simulink model "controller_template"  (Simulink 8.1)
settings: Solver=ode3  SolverMode=SingleTasking  StartTime=0.0  StopTime=inf  FixedStep=Ts  RelTol=1e-3
PreLoadFcn:
  | load_waypoints
values from neighbouring files (symbols this model uses):
  g = 9.8065    [kostas_malakies.mat]    (also in kostas_malakies2.mat; load_PMModel.m = 9.81; main.m; main_last.m)
  pitch_cmd2pitch_1stOrd = 1.42468924998    [kostas_malakies.mat]    (also in kostas_malakies2.mat)
  roll_cmd2roll_1stOrd = 1.38101661575    [kostas_malakies.mat]    (also in kostas_malakies2.mat)
  thrust_cmd2thrust_0thOrd = 0.876575459522    [kostas_malakies.mat]    (also in kostas_malakies2.mat)
  THRUST_CMD_GAIN = -0.0835    [kostas_malakies.mat]    (also in kostas_malakies2.mat; load_PMModel.m)
  yaw_cmd2yaw_1stOrd = 2.01792090263    [kostas_malakies.mat]    (also in kostas_malakies2.mat)
  z = [-0.93079906702 -0.933865725994 -0.937557637691 -0.939011216164 -0.94143640995 -0.944628417492 -0.947235524654 -0.949601888657 -0.952827751637 -0.9567258358 -0.958320975304 -0.960991024971 ... (7988 elements, 7988x1)]    [kostas_malakies2.mat]    (also in plotDataTest.m = simout_data.signals.values(:,11))
libraries: Hquad_control_LIB_MPC x3, simulink x1
settings Model: Creator=janosch  LastModifiedBy=burrimi  SimulationMode=external
settings DataIOCC: SaveOutput=off  SaveTime=off
settings OptimizationCC: OptimizeModelRefInitCode=on  LifeSpan=Inf
settings DebuggingCC: ParameterPrecisionLossMsg=none
settings HardwareCC: ProdIntDivRoundTo=Zero  ProdEndianess=LittleEndian  ProdHWDeviceType=Intel Pentium
settings RTWCC: SystemTargetFile=ert.tlc  TemplateMakefile=ert_default_tmf  Description=Embedded Coder  ProcessScript=ert_make_rtw_hook  CustomHeaderCode=#include <math.h>  TargetLang=C++  RTWCompilerOptimization=On
settings CodeAppCC: IgnoreCustomStorageClasses=off  CustomSymbolStrType=$N$R$M  InternalIdentifier=Classic
settings ERTTargetCC: CodeReplacementLibrary=ANSI_C  MultiwordLength=2048  GenerateSampleERTMain=on  SupportNonInlinedSFcns=on  ExtMode=on  ERTCustomFileTemplate=example_file_process.tlc  ConvertIfToSwitch=off  SuppressUnreachableDefaultCases=off
settings ConfigurationSet: Description=SimMechanics 2G

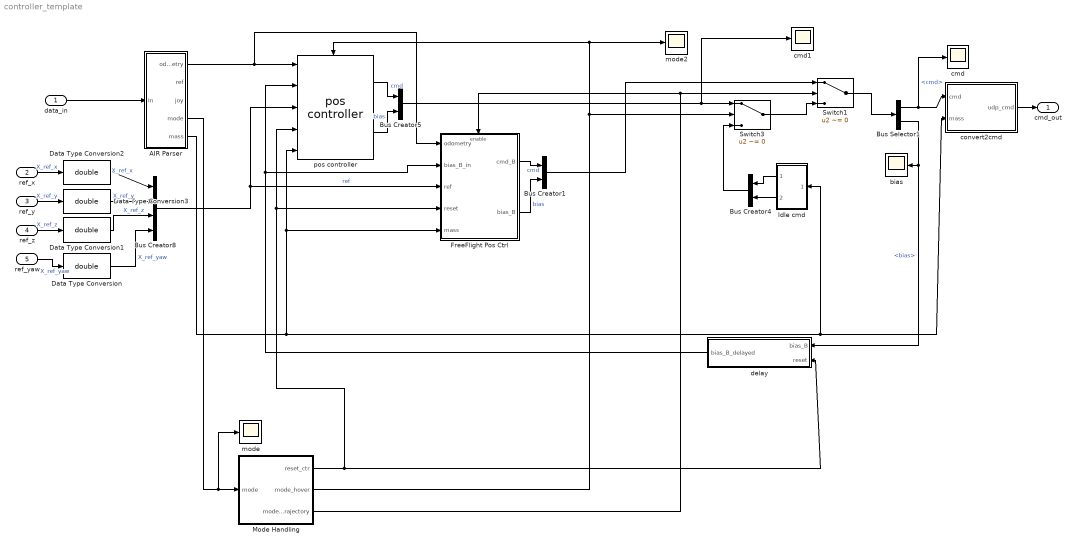
== system controller_template ==
  data_in : Inport  OutDataTypeStr=single  PortDimensions=30
  ref_x : Inport  Port=2  OutDataTypeStr=single  PortDimensions=93
  ref_y : Inport  Port=3  OutDataTypeStr=single  PortDimensions=93
  ref_z : Inport  Port=4  OutDataTypeStr=single  PortDimensions=62
  ref_yaw : Inport  Port=5  OutDataTypeStr=single  PortDimensions=62
  AIR Parser : Subsystem
  Bus Creator1 : BusCreator  Inputs=2
  Bus Creator4 : BusCreator  Inputs=2
  Bus Creator5 : BusCreator  Inputs=2
  Bus Creator8 : BusCreator
  Bus Selector1 : BusSelector  OutputSignals=cmd,bias
  Data Type Conversion{,1..3} (4 alike) : DataTypeConversion  OutDataTypeStr=double
  FreeFlight Pos Ctrl : Subsystem  AncestorBlock=Hquad_control_LIB_MPC/pos controller
  Idle cmd : Subsystem
  Mode Handling : Subsystem
  Switch1 : Switch  Criteria=u2 ~= 0
  Switch3 : Switch  Criteria=u2 ~= 0
  bias : Scope
      settings: TickLabels=on  TimeRange=40  YMin=-0.3  YMax=0.075  SaveName=ScopeData9
  cmd : Scope
      settings: YMin=-0.5  YMax=7  SaveName=ScopeData4
  cmd1 : Scope
      settings: YMin=-0.5  YMax=7  SaveName=ScopeData15
  convert2cmd : Subsystem
  delay : Subsystem
  mode : Scope
      settings: YMin=0  YMax=6  SaveName=ScopeData6
  mode2 : Scope
      settings: YMin=0  YMax=6  SaveName=ScopeData14
  pos controller : Hquad_control_LIB_MPC/pos controller
  cmd_out : Outport  PortDimensions=4
  wires:
  Mode Handling/1(reset_ctr) -> delay/2(reset), pos controller/4, FreeFlight Pos Ctrl/4(reset)
  Mode Handling/2(mode_hover) -> Switch3/2, mode2/1, pos controller/Enable
  AIR Parser/4(mode) -> mode/1, Mode Handling/1(mode)
  Bus Creator5/1 -> Switch3/1, cmd1/1
  pos controller/1 -> Bus Creator5/1  "cmd"
  pos controller/2 -> Bus Creator5/2  "bias"
  Bus Selector1/1 -> convert2cmd/1(cmd), cmd/1  "<cmd>"
  Bus Selector1/2 -> bias/1, delay/1(bias_B)  "<bias>"
  delay/1(bias_B_delayed) -> FreeFlight Pos Ctrl/2(bias_B_in), pos controller/2
  convert2cmd/1(udp_cmd) -> cmd_out/1
  data_in/1 -> AIR Parser/1(In)
  Idle cmd/1(cmd) -> Bus Creator4/1
  Idle cmd/2(bias) -> Bus Creator4/2
  Bus Creator4/1 -> Switch3/3
  AIR Parser/1(odometry) -> FreeFlight Pos Ctrl/1(odometry), pos controller/1
  ref_x/1 -> Data Type Conversion2/1  "X_ref_x"
  ref_y/1 -> Data Type Conversion3/1  "X_ref_y"
  ref_z/1 -> Data Type Conversion1/1  "X_ref_z"
  ref_yaw/1 -> Data Type Conversion/1  "X_ref_yaw"
  Data Type Conversion/1 -> Bus Creator8/4  "X_ref_yaw"
  Data Type Conversion1/1 -> Bus Creator8/3  "X_ref_z"
  Data Type Conversion2/1 -> Bus Creator8/1  "X_ref_x"
  Data Type Conversion3/1 -> Bus Creator8/2  "X_ref_y"
  Switch3/1 -> Switch1/3
  Switch1/1 -> Bus Selector1/1
  Mode Handling/3(mode_trajectory) -> FreeFlight Pos Ctrl/Enable, Switch1/2
  AIR Parser/5(mass) -> Idle cmd/1(mass), convert2cmd/2(mass), pos controller/5, FreeFlight Pos Ctrl/5(mass)
  Bus Creator8/1 -> pos controller/3, FreeFlight Pos Ctrl/3(ref)  "ref"
  Bus Creator1/1 -> Switch1/1
  FreeFlight Pos Ctrl/1(cmd_B) -> Bus Creator1/1  "cmd"
  FreeFlight Pos Ctrl/2(bias_B) -> Bus Creator1/2  "bias"

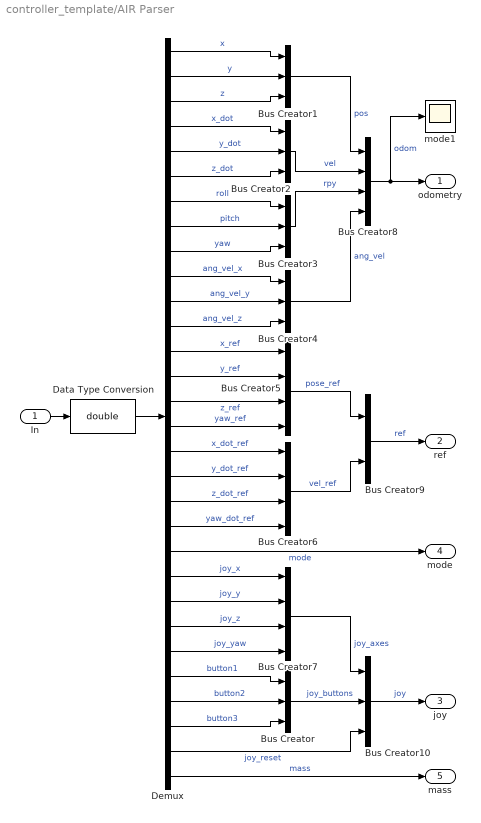
== system controller_template/AIR Parser ==
  In : Inport
  Bus Creator{,1..4,10} (6 alike) : BusCreator  Inputs=3
  Bus Creator{5..8} (4 alike) : BusCreator
  Bus Creator9 : BusCreator  Inputs=2
  Data Type Conversion : DataTypeConversion  OutDataTypeStr=double
  Demux : Demux  Outputs=30
  mode1 : Scope
      settings: YMin=0  YMax=6  SaveName=ScopeData7
  odometry : Outport
  ref : Outport  Port=2
  joy : Outport  Port=3
  mode : Outport  Port=4
  mass : Outport  Port=5
  wires:
  In/1 -> Data Type Conversion/1
  Data Type Conversion/1 -> Demux/1
  Demux/1 -> Bus Creator1/1  "x"
  Demux/7 -> Bus Creator3/1  "roll"
  Demux/8 -> Bus Creator3/2  "pitch"
  Demux/9 -> Bus Creator3/3  "yaw"
  Demux/15 -> Bus Creator5/3  "z_ref"
  Demux/14 -> Bus Creator5/2  "y_ref"
  Demux/13 -> Bus Creator5/1  "x_ref"
  Demux/16 -> Bus Creator5/4  "yaw_ref"
  Demux/2 -> Bus Creator1/2  "y"
  Demux/3 -> Bus Creator1/3  "z"
  Demux/4 -> Bus Creator2/1  "x_dot"
  Demux/5 -> Bus Creator2/2  "y_dot"
  Demux/6 -> Bus Creator2/3  "z_dot"
  Demux/19 -> Bus Creator6/3  "z_dot_ref"
  Demux/18 -> Bus Creator6/2  "y_dot_ref"
  Demux/17 -> Bus Creator6/1  "x_dot_ref"
  Demux/20 -> Bus Creator6/4  "yaw_dot_ref"
  Demux/12 -> Bus Creator4/3  "ang_vel_z"
  Demux/11 -> Bus Creator4/2  "ang_vel_y"
  Demux/10 -> Bus Creator4/1  "ang_vel_x"
  Demux/21 -> mode/1  "mode"
  Bus Creator5/1 -> Bus Creator9/1  "pose_ref"
  Bus Creator6/1 -> Bus Creator9/2  "vel_ref"
  Demux/22 -> Bus Creator7/1  "joy_x"
  Demux/23 -> Bus Creator7/2  "joy_y"
  Demux/24 -> Bus Creator7/3  "joy_z"
  Demux/25 -> Bus Creator7/4  "joy_yaw"
  Bus Creator7/1 -> Bus Creator10/1  "joy_axes"
  Demux/26 -> Bus Creator/1  "button1"
  Demux/28 -> Bus Creator/3  "button3"
  Demux/27 -> Bus Creator/2  "button2"
  Bus Creator/1 -> Bus Creator10/2  "joy_buttons"
  Bus Creator4/1 -> Bus Creator8/4  "ang_vel"
  Bus Creator3/1 -> Bus Creator8/3  "rpy"
  Bus Creator2/1 -> Bus Creator8/2  "vel"
  Bus Creator1/1 -> Bus Creator8/1  "pos"
  Demux/29 -> Bus Creator10/3  "joy_reset"
  Bus Creator10/1 -> joy/1  "joy"
  Bus Creator9/1 -> ref/1  "ref"
  Bus Creator8/1 -> odometry/1, mode1/1  "odom"
  Demux/30 -> mass/1  "mass"

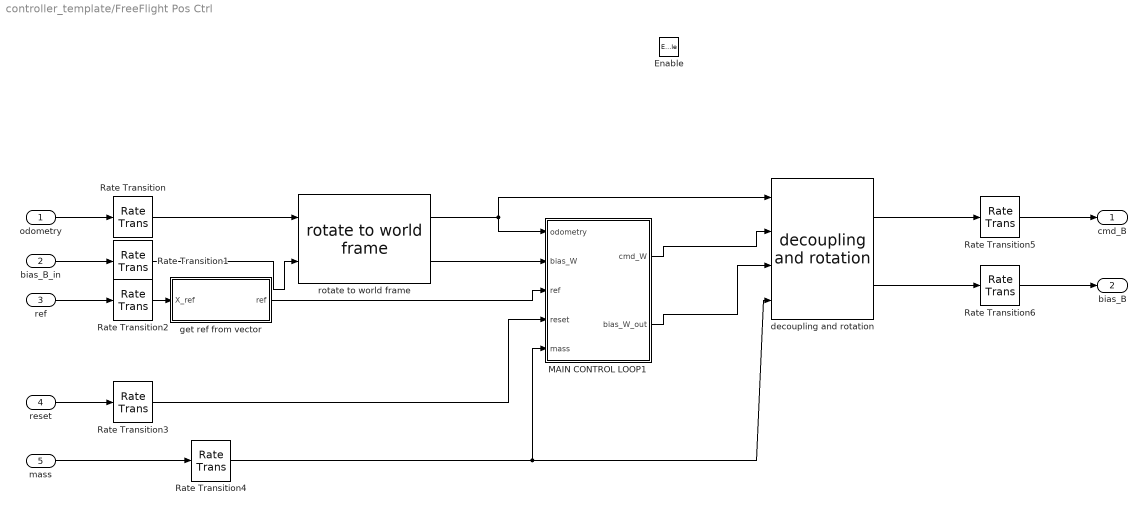
== system controller_template/FreeFlight Pos Ctrl ==
  odometry : Inport
  bias_B_in : Inport  Port=2
  ref : Inport  Port=3
  reset : Inport  Port=4
  mass : Inport  Port=5
  Enable : EnablePort  StatesWhenEnabling=reset
  MAIN CONTROL LOOP1 : Subsystem  Priority=2  AncestorBlock=Hquad_control_LIB_MPC/MAIN CONTROL LOOP  TreatAsAtomicUnit=on
  Rate Transition{,1..4} (5 alike) : RateTransition  OutPortSampleTime=0.08
  Rate Transition5 : RateTransition  OutPortSampleTime=Ts
  Rate Transition6 : RateTransition  OutPortSampleTime=Ts
  decoupling and rotation : Hquad_control_LIB_MPC/decoupling and rotation  Priority=3
  get ref from vector : Subsystem
  rotate to world frame : Hquad_control_LIB_MPC/rotate to world frame  Priority=1
  cmd_B : Outport
  bias_B : Outport  Port=2
  wires:
  mass/1 -> Rate Transition4/1
  bias_B_in/1 -> Rate Transition1/1
  rotate to world frame/2 -> MAIN CONTROL LOOP1/2(bias_W)
  decoupling and rotation/2 -> Rate Transition6/1
  decoupling and rotation/1 -> Rate Transition5/1
  MAIN CONTROL LOOP1/2(bias_W_out) -> decoupling and rotation/3
  rotate to world frame/1 -> decoupling and rotation/1, MAIN CONTROL LOOP1/1(odometry)
  ref/1 -> Rate Transition2/1
  reset/1 -> Rate Transition3/1
  MAIN CONTROL LOOP1/1(cmd_W) -> decoupling and rotation/2
  odometry/1 -> Rate Transition/1
  get ref from vector/1(ref) -> MAIN CONTROL LOOP1/3(ref)
  Rate Transition/1 -> rotate to world frame/1
  Rate Transition1/1 -> rotate to world frame/2
  Rate Transition2/1 -> get ref from vector/1(X_ref)
  Rate Transition3/1 -> MAIN CONTROL LOOP1/4(reset)
  Rate Transition4/1 -> decoupling and rotation/4, MAIN CONTROL LOOP1/5(mass)
  Rate Transition5/1 -> cmd_B/1
  Rate Transition6/1 -> bias_B/1

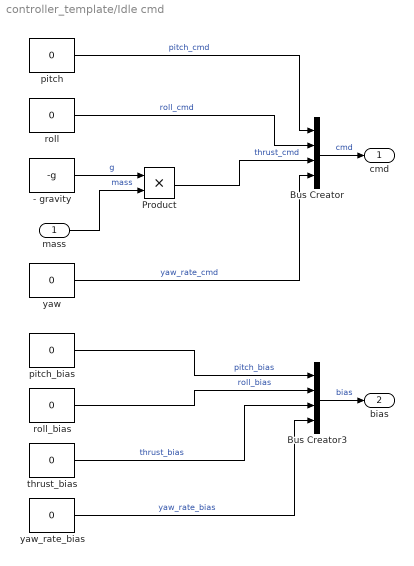
== system controller_template/Idle cmd ==
  mass : Inport  OutDataTypeStr=double
  - gravity : Constant  Value=-g
  Bus Creator : BusCreator
  Bus Creator3 : BusCreator
  Product : Product  RndMeth=Zero
  pitch : Constant  Value=0
  pitch_bias : Constant  Value=0
  roll : Constant  Value=0
  roll_bias : Constant  Value=0
  thrust_bias : Constant  Value=0
  yaw : Constant  Value=0
  yaw_rate_bias : Constant  Value=0
  cmd : Outport
  bias : Outport  Port=2
  wires:
  roll/1 -> Bus Creator/2  "roll_cmd"
  pitch/1 -> Bus Creator/1  "pitch_cmd"
  Bus Creator/1 -> cmd/1  "cmd"
  yaw/1 -> Bus Creator/4  "yaw_rate_cmd"
  pitch_bias/1 -> Bus Creator3/1  "pitch_bias"
  roll_bias/1 -> Bus Creator3/2  "roll_bias"
  thrust_bias/1 -> Bus Creator3/3  "thrust_bias"
  yaw_rate_bias/1 -> Bus Creator3/4  "yaw_rate_bias"
  Bus Creator3/1 -> bias/1  "bias"
  - gravity/1 -> Product/1  "g"
  Product/1 -> Bus Creator/3  "thrust_cmd"
  mass/1 -> Product/2  "mass"

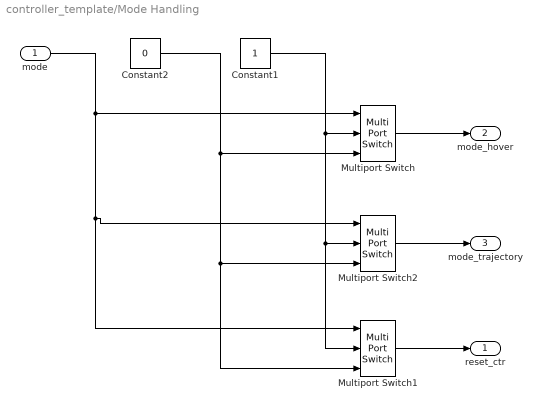
== system controller_template/Mode Handling ==
  mode : Inport
  Constant1 : Constant
  Constant2 : Constant  Value=0
  Multiport Switch : MultiPortSwitch  DataPortOrder=Specify indices  Inputs=2  DataPortIndices={[1,2,3],0}
  Multiport Switch1 : MultiPortSwitch  DataPortOrder=Specify indices  Inputs=2  DataPortIndices={[10],0}
  Multiport Switch2 : MultiPortSwitch  DataPortOrder=Specify indices  Inputs=2  DataPortIndices={[4],0}
  reset_ctr : Outport
  mode_hover : Outport  Port=2
  mode_trajectory : Outport  Port=3
  wires:
  Constant1/1 -> Multiport Switch/2, Multiport Switch1/2, Multiport Switch2/2
  Constant2/1 -> Multiport Switch/3, Multiport Switch1/3, Multiport Switch2/3
  Multiport Switch1/1 -> reset_ctr/1
  mode/1 -> Multiport Switch/1, Multiport Switch1/1, Multiport Switch2/1
  Multiport Switch/1 -> mode_hover/1
  Multiport Switch2/1 -> mode_trajectory/1

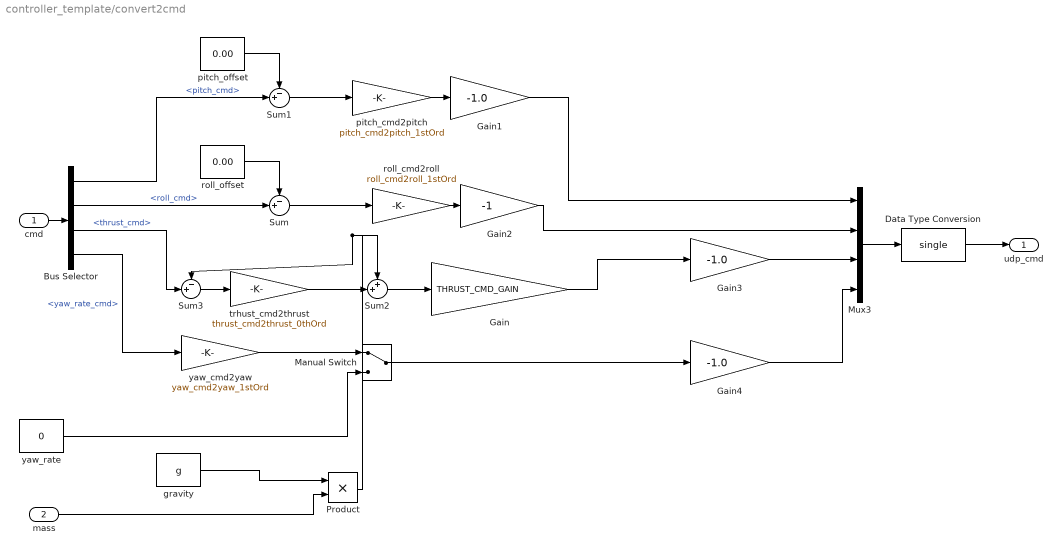
== system controller_template/convert2cmd ==
  cmd : Inport
  mass : Inport  Port=2
  Bus Selector : BusSelector  OutputSignals=pitch_cmd,roll_cmd,thrust_cmd,yaw_rate_cmd
  Data Type Conversion : DataTypeConversion  OutDataTypeStr=single
  Gain : Gain  Gain=THRUST_CMD_GAIN
  Gain1 : Gain  Gain=-1.0
  Gain2 : Gain  Gain=-1
  Gain3 : Gain  Gain=-1.0
  Gain4 : Gain  Gain=-1.0
  Manual Switch : ManualSwitch
  Mux3 : Mux
  Product : Product  RndMeth=Zero
  Sum : Sum  Inputs=-+|
  Sum1 : Sum  Inputs=-+|
  Sum2 : Sum  Inputs=++|
  Sum3 : Sum  Inputs=-+|
  gravity : Constant  Value=g
  pitch_cmd2pitch : Gain  Gain=pitch_cmd2pitch_1stOrd
  pitch_offset : Constant  Value=0.00
  roll_cmd2roll : Gain  Gain=roll_cmd2roll_1stOrd
  roll_offset : Constant  Value=0.00
  trhust_cmd2thrust : Gain  Gain=thrust_cmd2thrust_0thOrd
  yaw_cmd2yaw : Gain  Gain=yaw_cmd2yaw_1stOrd
  yaw_rate : Constant  Value=0
  udp_cmd : Outport
  wires:
  pitch_cmd2pitch/1 -> Gain1/1
  Bus Selector/2 -> Sum/2  "<roll_cmd>"
  Sum/1 -> roll_cmd2roll/1
  roll_offset/1 -> Sum/1
  Gain4/1 -> Mux3/4
  Gain3/1 -> Mux3/3
  Gain2/1 -> Mux3/2
  Gain/1 -> Gain3/1
  Gain1/1 -> Mux3/1
  pitch_offset/1 -> Sum1/1
  Sum1/1 -> pitch_cmd2pitch/1
  Mux3/1 -> Data Type Conversion/1
  Data Type Conversion/1 -> udp_cmd/1
  Product/1 -> Sum2/1, Sum3/1
  Sum2/1 -> Gain/1
  Manual Switch/1 -> Gain4/1
  yaw_rate/1 -> Manual Switch/2
  cmd/1 -> Bus Selector/1
  Bus Selector/1 -> Sum1/2  "<pitch_cmd>"
  yaw_cmd2yaw/1 -> Manual Switch/1
  trhust_cmd2thrust/1 -> Sum2/2
  roll_cmd2roll/1 -> Gain2/1
  Bus Selector/3 -> Sum3/2  "<thrust_cmd>"
  Sum3/1 -> trhust_cmd2thrust/1
  Bus Selector/4 -> yaw_cmd2yaw/1  "<yaw_rate_cmd>"
  gravity/1 -> Product/1
  mass/1 -> Product/2

== system controller_template/delay ==
  bias_B : Inport
  reset : Inport  Port=2
  Bus Creator1 : BusCreator
  Demux1 : Demux
  delay bias : simulink/Additional Math & Discrete/Additional Discrete/Unit Delay Resettable  vinit=0.0  tsamp=-1
  bias_B_delayed : Outport
  wires:
  Demux1/1 -> Bus Creator1/1  "pitch_bias"
  Demux1/2 -> Bus Creator1/2  "roll_bias"
  Demux1/3 -> Bus Creator1/3  "thrust_bias"
  Demux1/4 -> Bus Creator1/4  "yaw_rate_bias"
  delay bias/1 -> Demux1/1
  bias_B/1 -> delay bias/1
  reset/1 -> delay bias/2
  Bus Creator1/1 -> bias_B_delayed/1

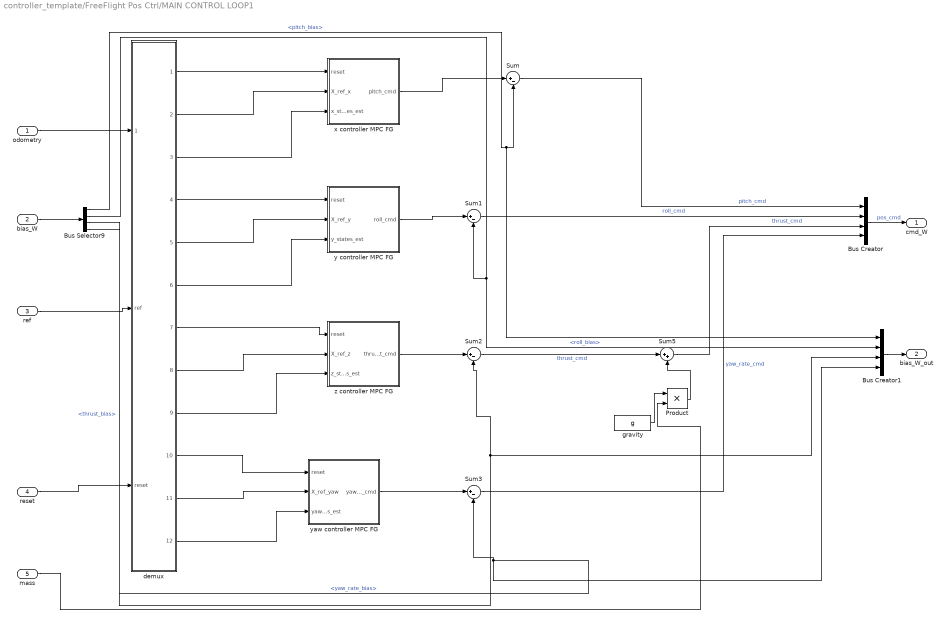
== system controller_template/FreeFlight Pos Ctrl/MAIN CONTROL LOOP1 ==
  odometry : Inport
  bias_W : Inport  Port=2
  ref : Inport  Port=3
  reset : Inport  Port=4
  mass : Inport  Port=5
  Bus Creator : BusCreator
  Bus Creator1 : BusCreator
  Bus Selector9 : BusSelector  OutputSignals=pitch_bias,roll_bias,thrust_bias,yaw_rate_bias
  Product : Product  RndMeth=Zero
  Sum{,1..3} (4 alike) : Sum  Inputs=|+-
  Sum5 : Sum  Inputs=|++
  demux : Subsystem
  gravity : Constant  Value=g
  "x controller MPC FG  " : Subsystem  AncestorBlock=Hquad_control_LIB_MPC/x controller MPC FG
  y controller MPC FG : Subsystem  AncestorBlock=Hquad_control_LIB_MPC/y controller MPC FG
  yaw controller MPC FG : Subsystem  AncestorBlock=Hquad_control_LIB_MPC/yaw controller MPC FG
  z controller MPC FG : Subsystem  AncestorBlock=Hquad_control_LIB_MPC/z controller MPC FG
  cmd_W : Outport
  bias_W_out : Outport  Port=2
  wires:
  Bus Selector9/4 -> Sum3/2, Bus Creator1/4  "<yaw_rate_bias>"
  Sum3/1 -> Bus Creator/4  "yaw_rate_cmd"
  Bus Selector9/3 -> Sum2/2, Bus Creator1/3  "<thrust_bias>"
  Bus Selector9/1 -> Sum/2, Bus Creator1/1  "<pitch_bias>"
  Bus Selector9/2 -> Bus Creator1/2, Sum1/2  "<roll_bias>"
  bias_W/1 -> Bus Selector9/1
  Sum5/1 -> Bus Creator/3  "thrust_cmd"
  Bus Creator1/1 -> bias_W_out/1
  Sum2/1 -> Sum5/1  "thrust_cmd"
  Sum1/1 -> Bus Creator/2  "roll_cmd"
  Sum/1 -> Bus Creator/1  "pitch_cmd"
  odometry/1 -> demux/1(odometry)
  ref/1 -> demux/2(ref)
  reset/1 -> demux/3(reset)
  demux/1(reset1) -> "x controller MPC FG  "/1(reset)
  demux/4(reset2) -> y controller MPC FG/1(reset)
  demux/7(reset3) -> z controller MPC FG/1(reset)
  demux/10(reset4) -> yaw controller MPC FG/1(reset)
  Bus Creator/1 -> cmd_W/1  "pos_cmd"
  mass/1 -> Product/2
  Product/1 -> Sum5/2
  gravity/1 -> Product/1
  "x controller MPC FG  "/1("pitch_cmd   ") -> Sum/1
  y controller MPC FG/1(roll_cmd) -> Sum1/1
  z controller MPC FG/1(thrust_cmd) -> Sum2/1
  yaw controller MPC FG/1(yaw_rate_cmd) -> Sum3/1
  demux/2(X_ref_x) -> "x controller MPC FG  "/2("X_ref_x  ")
  demux/3(x_states) -> "x controller MPC FG  "/3("x_states_est  ")
  demux/5(X_ref_y) -> y controller MPC FG/2("X_ref_y  ")
  demux/6(y_states) -> y controller MPC FG/3("y_states_est  ")
  demux/8(X_ref_z) -> z controller MPC FG/2(X_ref_z)
  demux/9(z_states) -> z controller MPC FG/3("z_states_est  ")
  demux/11(X_ref_yaw) -> yaw controller MPC FG/2(X_ref_yaw)
  demux/12(yaw_states) -> yaw controller MPC FG/3("yaw_states_est  ")

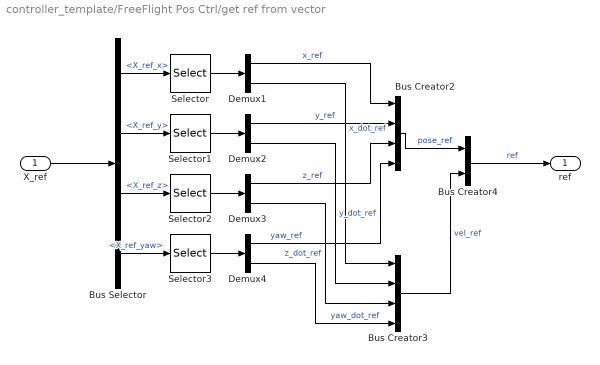
== system controller_template/FreeFlight Pos Ctrl/get ref from vector ==
  X_ref : Inport
  Bus Creator2 : BusCreator
  Bus Creator3 : BusCreator
  Bus Creator4 : BusCreator  Inputs=2
  Bus Selector : BusSelector  OutputSignals=X_ref_x,X_ref_y,X_ref_z,X_ref_yaw
  Demux{1..4} (4 alike) : Demux  Outputs=2
  Selector{,1..3} (4 alike) : Selector  IndexOptions=Index vector (dialog)  Indices=[1 2]  OutputSizes=1
  ref : Outport
  wires:
  X_ref/1 -> Bus Selector/1
  Bus Selector/1 -> Selector/1  "<X_ref_x>"
  Bus Selector/4 -> Selector3/1  "<X_ref_yaw>"
  Bus Selector/3 -> Selector2/1  "<X_ref_z>"
  Bus Selector/2 -> Selector1/1  "<X_ref_y>"
  Selector/1 -> Demux1/1
  Selector3/1 -> Demux4/1
  Selector2/1 -> Demux3/1
  Selector1/1 -> Demux2/1
  Bus Creator2/1 -> Bus Creator4/1  "pose_ref"
  Bus Creator3/1 -> Bus Creator4/2  "vel_ref"
  Bus Creator4/1 -> ref/1  "ref"
  Demux1/1 -> Bus Creator2/1  "x_ref"
  Demux2/1 -> Bus Creator2/2  "y_ref"
  Demux3/1 -> Bus Creator2/3  "z_ref"
  Demux4/1 -> Bus Creator2/4  "yaw_ref"
  Demux1/2 -> Bus Creator3/1  "x_dot_ref"
  Demux2/2 -> Bus Creator3/2  "y_dot_ref"
  Demux3/2 -> Bus Creator3/3  "z_dot_ref"
  Demux4/2 -> Bus Creator3/4  "yaw_dot_ref"

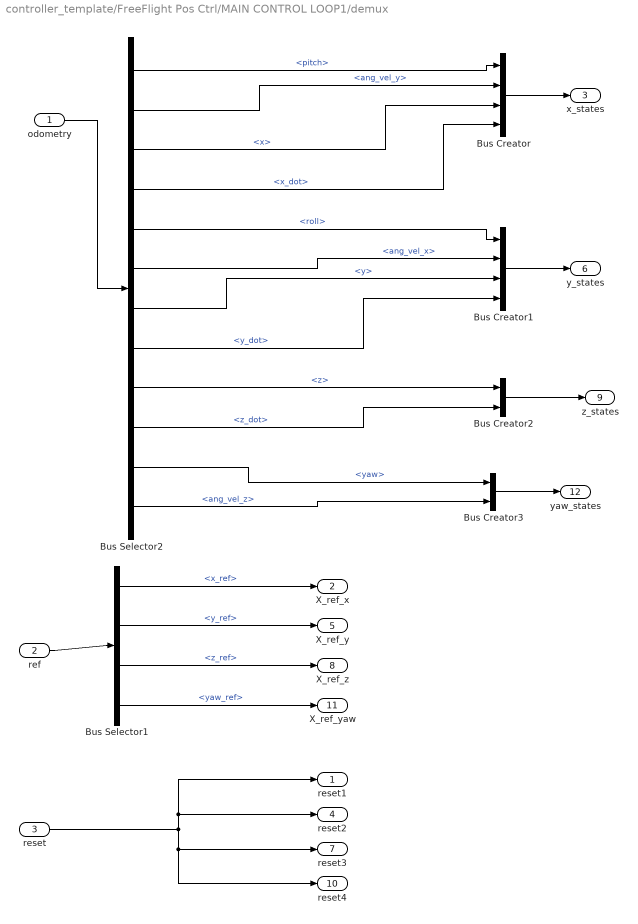
== system controller_template/FreeFlight Pos Ctrl/MAIN CONTROL LOOP1/demux ==
  odometry : Inport
  ref : Inport  Port=2
  reset : Inport  Port=3
  Bus Creator : BusCreator
  Bus Creator1 : BusCreator
  Bus Creator2 : BusCreator  Inputs=2
  Bus Creator3 : BusCreator  Inputs=2
  Bus Selector1 : BusSelector  OutputSignals=pose_ref.x_ref,pose_ref.y_ref,pose_ref.z_ref,pose_ref.yaw_ref
  Bus Selector2 : BusSelector  OutputSignals=rpy.pitch,ang_vel.ang_vel_y,pos.x,vel.x_dot,rpy.roll,ang_vel.ang_vel_x,pos.y,vel.y_dot,pos.z,vel.z_dot,rpy.yaw,ang_vel.ang_vel_z
  reset1 : Outport
  X_ref_x : Outport  Port=2
  x_states : Outport  Port=3
  reset2 : Outport  Port=4
  X_ref_y : Outport  Port=5
  y_states : Outport  Port=6
  reset3 : Outport  Port=7
  X_ref_z : Outport  Port=8
  z_states : Outport  Port=9
  reset4 : Outport  Port=10
  X_ref_yaw : Outport  Port=11
  yaw_states : Outport  Port=12
  wires:
  Bus Selector1/4 -> X_ref_yaw/1  "<yaw_ref>"
  Bus Selector1/3 -> X_ref_z/1  "<z_ref>"
  odometry/1 -> Bus Selector2/1
  ref/1 -> Bus Selector1/1
  Bus Selector1/1 -> X_ref_x/1  "<x_ref>"
  Bus Selector1/2 -> X_ref_y/1  "<y_ref>"
  reset/1 -> reset3/1, reset4/1, reset2/1, reset1/1
  Bus Creator/1 -> x_states/1
  Bus Selector2/1 -> Bus Creator/1  "<pitch>"
  Bus Selector2/2 -> Bus Creator/2  "<ang_vel_y>"
  Bus Selector2/3 -> Bus Creator/3  "<x>"
  Bus Selector2/4 -> Bus Creator/4  "<x_dot>"
  Bus Creator1/1 -> y_states/1
  Bus Selector2/5 -> Bus Creator1/1  "<roll>"
  Bus Selector2/6 -> Bus Creator1/2  "<ang_vel_x>"
  Bus Selector2/7 -> Bus Creator1/3  "<y>"
  Bus Selector2/8 -> Bus Creator1/4  "<y_dot>"
  Bus Selector2/9 -> Bus Creator2/1  "<z>"
  Bus Selector2/10 -> Bus Creator2/2  "<z_dot>"
  Bus Selector2/12 -> Bus Creator3/2  "<ang_vel_z>"
  Bus Selector2/11 -> Bus Creator3/1  "<yaw>"
  Bus Creator2/1 -> z_states/1
  Bus Creator3/1 -> yaw_states/1

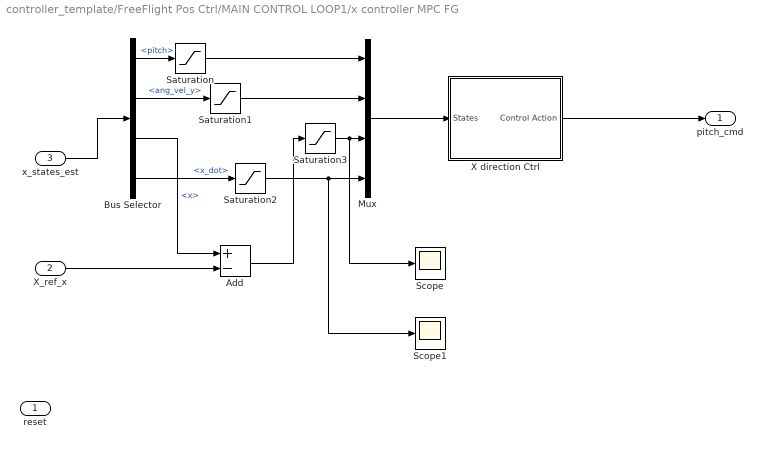
== system controller_template/FreeFlight Pos Ctrl/MAIN CONTROL LOOP1/x controller MPC FG   ==
  reset : Inport  PortDimensions=1
  "X_ref_x  " : Inport  Port=2
  "x_states_est  " : Inport  Port=3
  Add : Sum  Inputs=+-
  Bus Selector : BusSelector  OutputSignals=pitch,ang_vel_y,x,x_dot
  Mux : Mux
  Saturation : Saturate  UpperLimit=0.2094  LowerLimit=-0.2094
  Saturation1 : Saturate  UpperLimit=2  LowerLimit=-2
  Saturation2 : Saturate  UpperLimit=1  LowerLimit=-1
  Saturation3 : Saturate  UpperLimit=1  LowerLimit=-1
  Scope : Scope
      settings: SaveName=ScopeData11
  Scope1 : Scope
      settings: SaveName=ScopeData12
  X direction Ctrl : Subsystem  AncestorBlock=mpt_sim/Explicit Controller  mask(MPT Controller){}
      mask help: Evaluates explicit controller for a given state.
      mask Help: Evaluation of an explicit control law is performed by the C-code S-function "mpt_getInput_sfunc", which requires the controller to be exported to C-code using "exportToC".
      mask Display: image(imread('mpt_ctrl.jpg'));
  "pitch_cmd   " : Outport  PortDimensions=1
  wires:
  X direction Ctrl/1(Control Action) -> "pitch_cmd   "/1
  "X_ref_x  "/1 -> Add/2
  Bus Selector/1 -> Saturation/1  "<pitch>"
  Bus Selector/2 -> Saturation1/1  "<ang_vel_y>"
  Bus Selector/3 -> Add/1  "<x>"
  Add/1 -> Saturation3/1
  Bus Selector/4 -> Saturation2/1  "<x_dot>"
  Mux/1 -> X direction Ctrl/1(States)
  "x_states_est  "/1 -> Bus Selector/1
  Saturation/1 -> Mux/1
  Saturation1/1 -> Mux/2
  Saturation2/1 -> Scope1/1, Mux/4
  Saturation3/1 -> Scope/1, Mux/3

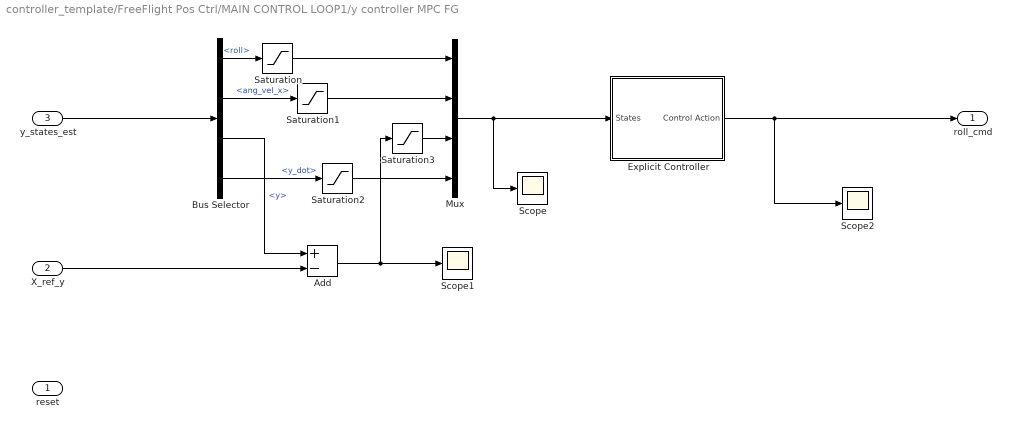
== system controller_template/FreeFlight Pos Ctrl/MAIN CONTROL LOOP1/y controller MPC FG ==
  reset : Inport  PortDimensions=1
  "X_ref_y  " : Inport  Port=2
  "y_states_est  " : Inport  Port=3
  Add : Sum  Inputs=+-
  Bus Selector : BusSelector  OutputSignals=roll,ang_vel_x,y,y_dot
  Explicit Controller : Subsystem  AncestorBlock=mpt_sim/Explicit Controller  mask(MPT Controller){}
      mask help: Evaluates explicit controller for a given state.
      mask Help: Evaluation of an explicit control law is performed by the C-code S-function "mpt_getInput_sfunc", which requires the controller to be exported to C-code using "exportToC".
      mask Display: image(imread('mpt_ctrl.jpg'));
  Mux : Mux
  Saturation : Saturate  UpperLimit=0.2094  LowerLimit=-0.2094
  Saturation1 : Saturate  UpperLimit=2  LowerLimit=-2
  Saturation2 : Saturate  UpperLimit=1  LowerLimit=-1
  Saturation3 : Saturate  UpperLimit=1  LowerLimit=-1
  Scope : Scope
      settings: SaveName=ScopeData3
  Scope1 : Scope
      settings: SaveName=ScopeData5
  Scope2 : Scope
      settings: SaveName=ScopeData6
  roll_cmd : Outport  PortDimensions=1
  wires:
  Explicit Controller/1(Control Action) -> Scope2/1, roll_cmd/1
  "X_ref_y  "/1 -> Add/2
  Bus Selector/1 -> Saturation/1  "<roll>"
  Bus Selector/2 -> Saturation1/1  "<ang_vel_x>"
  Bus Selector/3 -> Add/1  "<y>"
  Add/1 -> Scope1/1, Saturation3/1
  Bus Selector/4 -> Saturation2/1  "<y_dot>"
  Mux/1 -> Scope/1, Explicit Controller/1(States)
  "y_states_est  "/1 -> Bus Selector/1
  Saturation/1 -> Mux/1
  Saturation1/1 -> Mux/2
  Saturation2/1 -> Mux/4
  Saturation3/1 -> Mux/3

== system controller_template/FreeFlight Pos Ctrl/MAIN CONTROL LOOP1/yaw controller MPC FG ==
  reset : Inport  PortDimensions=1
  X_ref_yaw : Inport  Port=2
  "yaw_states_est  " : Inport  Port=3
  Add : Sum  Inputs=+-
  Demux : Demux  Outputs=2
  Explicit Controller : Subsystem  AncestorBlock=mpt_sim/Explicit Controller  mask(MPT Controller){}
      mask help: Evaluates explicit controller for a given state.
      mask Help: Evaluation of an explicit control law is performed by the C-code S-function "mpt_getInput_sfunc", which requires the controller to be exported to C-code using "exportToC".
      mask Display: image(imread('mpt_ctrl.jpg'));
  Saturation : Saturate  UpperLimit=0.0873  LowerLimit=-0.0873
  yaw_rate_cmd : Outport  PortDimensions=1
  wires:
  X_ref_yaw/1 -> Add/2
  "yaw_states_est  "/1 -> Demux/1
  Demux/1 -> Add/1
  Add/1 -> Saturation/1
  Explicit Controller/1(Control Action) -> yaw_rate_cmd/1
  Saturation/1 -> Explicit Controller/1(States)

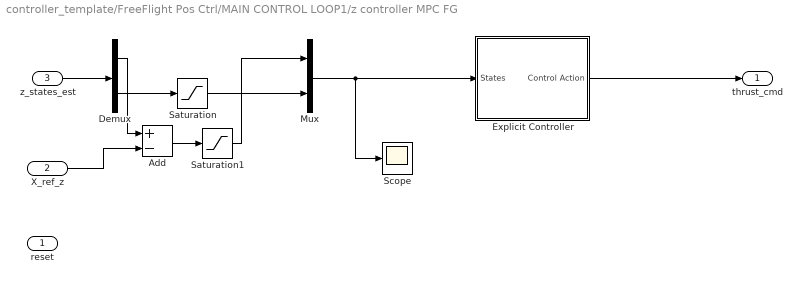
== system controller_template/FreeFlight Pos Ctrl/MAIN CONTROL LOOP1/z controller MPC FG ==
  reset : Inport  PortDimensions=1
  X_ref_z : Inport  Port=2
  "z_states_est  " : Inport  Port=3
  Add : Sum  Inputs=+-
  Demux : Demux  Outputs=2
  Explicit Controller : Subsystem  AncestorBlock=mpt_sim/Explicit Controller  mask(MPT Controller){}
      mask help: Evaluates explicit controller for a given state.
      mask Help: Evaluation of an explicit control law is performed by the C-code S-function "mpt_getInput_sfunc", which requires the controller to be exported to C-code using "exportToC".
      mask Display: image(imread('mpt_ctrl.jpg'));
  Mux : Mux  Inputs=2
  Saturation : Saturate  UpperLimit=1  LowerLimit=-1
  Saturation1 : Saturate  UpperLimit=1  LowerLimit=-1
  Scope : Scope
      settings: SaveName=ScopeData2
  thrust_cmd : Outport  PortDimensions=1
  wires:
  "z_states_est  "/1 -> Demux/1
  Demux/2 -> Saturation/1
  Demux/1 -> Add/1
  X_ref_z/1 -> Add/2
  Add/1 -> Saturation1/1
  Explicit Controller/1(Control Action) -> thrust_cmd/1
  Mux/1 -> Scope/1, Explicit Controller/1(States)
  Saturation/1 -> Mux/2
  Saturation1/1 -> Mux/1

== system controller_template/FreeFlight Pos Ctrl/MAIN CONTROL LOOP1/x controller MPC FG  /X direction Ctrl ==
  States : Inport
  MATLAB Function : MATLAB Function  TreatAsAtomicUnit=on
  S-Function : S-Function  FunctionName=mpt_getInput_sfunc_XdirectionFF  EnableBusSupport=off
  Control Action : Outport
  wires:
  S-Function/1 -> Control Action/1
  States/1 -> S-Function/1

== system controller_template/FreeFlight Pos Ctrl/MAIN CONTROL LOOP1/y controller MPC FG/Explicit Controller ==
  States : Inport
  S-Function : S-Function  FunctionName=mpt_getInput_sfunc_Ydirection  EnableBusSupport=off
  Control Action : Outport
  wires:
  S-Function/1 -> Control Action/1
  States/1 -> S-Function/1

== system controller_template/FreeFlight Pos Ctrl/MAIN CONTROL LOOP1/yaw controller MPC FG/Explicit Controller ==
  States : Inport
  S-Function : S-Function  FunctionName=mpt_getInput_sfunc_YawCtrl  EnableBusSupport=off
  Control Action : Outport
  wires:
  S-Function/1 -> Control Action/1
  States/1 -> S-Function/1

== system controller_template/FreeFlight Pos Ctrl/MAIN CONTROL LOOP1/z controller MPC FG/Explicit Controller ==
  States : Inport
  S-Function : S-Function  FunctionName=mpt_getInput_sfunc_Zdirection  EnableBusSupport=off
  Control Action : Outport
  wires:
  S-Function/1 -> Control Action/1
  States/1 -> S-Function/1

== matlab function FreeFlight Pos Ctrl/MAIN CONTROL LOOP1/x controller MPC FG /X direction Ctrl/MATLAB Function ==
  data: u input double; y output double
function y = fcn(u)
%#codegen

y = u;
